simulink model "InvertPendLinearPlantControl"  (R2022b)
settings: Solver=VariableStepAuto  StartTime=0.0  StopTime=10.0  RelTol=1e-6  AbsTol=1e-6
PreLoadFcn:
  | init_condLinPlant
  | load('K1.mat')
values from neighbouring files (symbols this model uses):
  A = [0 1 0 0; (M*g + g*m)/(M*l) -d 0 0; 0 0 0 1; (g*m)/M 0 0 -d]    [init_condLQG.m]    (also in init_condLinPlant.m)
  B = [0; 1/(M*l); 0; 1/M]    [init_condLQG.m]    (also in init_condLinPlant.m)
  C = [1 0 0 0; 0 0 1 0]    [init_condLQG.m]    (also in init_condLinPlant.m = [0 0 1 0])
  D = [0; 0]    [init_condLQG.m]    (also in init_condLinPlant.m = 0)
  K = [152.357859327 61.9938837921 -2.44892966361 -6.99694189604]    [K1.mat]    (also in K2.mat = [274.714705787 116.856004488 -14.1421356237 -23.6448310047])
  N = .001*ones(4,1)    [init_condLinPlant.m]
  R = [0.0125;0.7620]    [init_condLQG.m]    (also in init_condLinPlant.m = 0.8277)
undefined symbols (not defined in the file or in its folder): Continuous, Time
libraries: simulink_extras x2, ctrlSharedLib x1
settings Model: Creator=antsupove  LastModifiedBy=antsupove

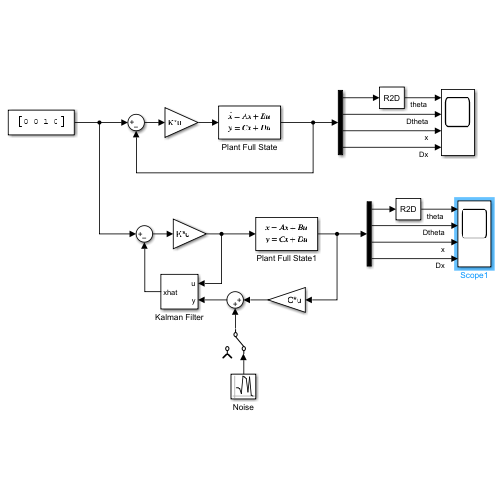
[thumbnail: Simulink's stored preview of the top-level diagram]
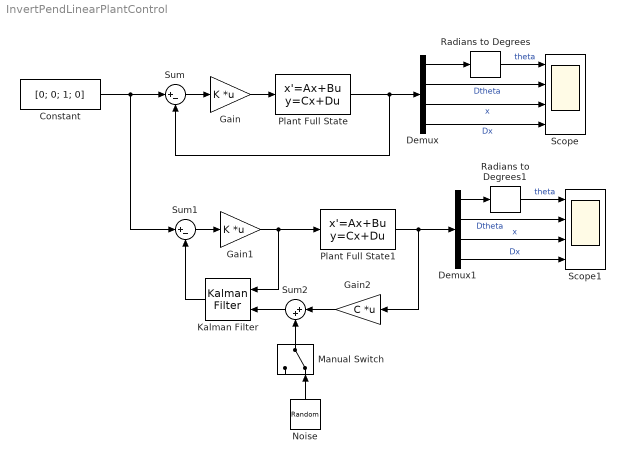
== system InvertPendLinearPlantControl ==
  Constant : Constant  Value=[0; 0; 1; 0]
  Demux : Demux
  Demux1 : Demux
  Gain : Gain  Gain=K  Multiplication=Matrix(K*u)
  Gain1 : Gain  Gain=K  Multiplication=Matrix(K*u)
  Gain2 : Gain  Gain=C  Multiplication=Matrix(K*u)
  Kalman Filter : ctrlSharedLib/Kalman Filter  TimeDomain=Continuous-Time  UseCurrentEstimator=on  ModelSource=Individual A, B, C, D matrices  ModelSourceVariable=ss(0.95,1,1,0,1)  A=A  B=B  C=C  D=D  NumberOfStates=1  NumberOfInputs=1  NumberOfOutputs=1  InitialEstimateSource=Dialog  X0=0  P0=10  UseK=off  UseGH=on  NumberOfProcessNoiseInputs=1  G=G  TimeInvariantG=on  H=H  TimeInvariantH=on  Q=Q  TimeInvariantQ=on  R=R  TimeInvariantR=on  N=N  TimeInvariantN=on  AddInputPort=on  AddEnablePort=off  OutputEstimatedY=off  OutputP=off  Ts=-1
  Manual Switch : ManualSwitch  CurrentSetting=0
  Noise : RandomNumber  Variance=.0001  Seed=1  SampleTime=0.01
  Plant Full State : StateSpace  A=A  B=B  C=eye(4)  D=[0; 0; 0; 0]  InitialCondition=0
  Plant Full State1 : StateSpace  A=A  B=B  C=eye(4)  D=[0; 0; 0; 0]  InitialCondition=0
  Radians to Degrees : simulink_extras/Transformations/Radians to Degrees
  Radians to Degrees1 : simulink_extras/Transformations/Radians to Degrees
  Scope : Scope  NumInputPorts=4
  Scope1 : Scope  NumInputPorts=4
  Sum : Sum  Inputs=|+-
  Sum1 : Sum  Inputs=|+-
  Sum2 : Sum  Inputs=|++
  wires:
  Plant Full State/1 -> Sum/2, Demux/1
  Constant/1 -> Sum/1, Sum1/1
  Sum/1 -> Gain/1
  Gain/1 -> Plant Full State/1
  Demux/1 -> Radians to Degrees/1
  Demux/2 -> Scope/2  "Dtheta"
  Demux/3 -> Scope/3  "x"
  Demux/4 -> Scope/4  "Dx"
  Radians to Degrees/1 -> Scope/1  "theta"
  Gain1/1 -> Plant Full State1/1, Kalman Filter/1
  Sum1/1 -> Gain1/1
  Kalman Filter/1 -> Sum1/2
  Plant Full State1/1 -> Gain2/1, Demux1/1
  Radians to Degrees1/1 -> Scope1/1  "theta"
  Demux1/4 -> Scope1/4  "Dx"
  Demux1/3 -> Scope1/3  "x"
  Demux1/2 -> Scope1/2  "Dtheta"
  Demux1/1 -> Radians to Degrees1/1
  Gain2/1 -> Sum2/1
  Sum2/1 -> Kalman Filter/2
  Manual Switch/1 -> Sum2/2
  Noise/1 -> Manual Switch/2
